simulink model "TestController"  (R2022b)
settings: Solver=FixedStepAuto  StartTime=0.0  StopTime=10.0  RelTol=1e-3
settings Model: Creator=hollis  LastModifiedBy=hollis
settings OptimizationCC: DefaultParameterBehavior=Inlined  EnhancedBackFolding=on  PassReuseOutputArgsAs=Individual arguments  ZeroExternalMemoryAtStartup=off  ZeroInternalMemoryAtStartup=off  OptimizeBlockOrder=speed  DifferentSizesBufferReuse=on  OptimizationCustomize=off  EfficientTunableParamExpr=on
settings DebuggingCC: ParameterTunabilityLossMsg=error
settings SFSimCC: MATLABDynamicMemAlloc=off
settings RTWCC: Description=Embedded Coder  SystemTargetFile=ert.tlc  TemplateMakefile=ert_default_tmf  TargetLang=C++
settings CodeAppCC: ForceParamTrailComments=on  IgnoreCustomStorageClasses=off  OperatorAnnotations=on  SimulinkDataObjDesc=on  SFDataObjDesc=on  InsertBlockDesc=on
settings ERTTargetCC: TargetLangStandard=C++11 (ISO)  GenerateSampleERTMain=on  CodeInterfacePackaging=C++ class  SupportContinuousTime=on  InlinedParameterPlacement=NonHierarchical  RootIOFormat=Structure reference  ERTCustomFileTemplate=example_file_process.tlc

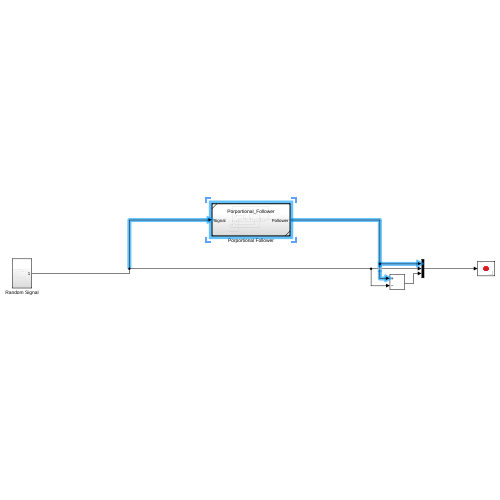
[thumbnail: Simulink's stored preview of the top-level diagram]
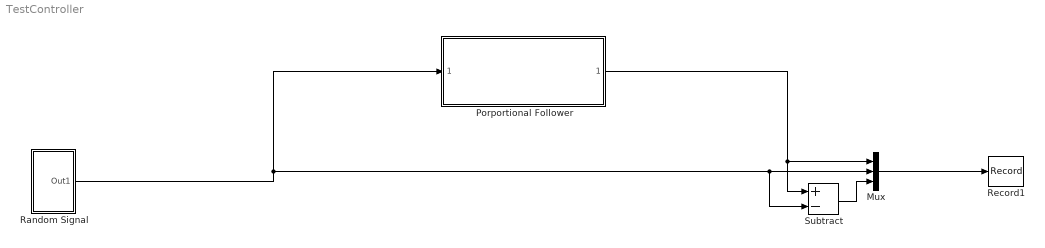
== system TestController ==
  Mux : Mux  Inputs=3
  Porportional Follower : Subsystem  TreatAsAtomicUnit=on  ReferencedSubsystem=Porportional_Follower
  Random Signal : Subsystem
  Record1 : Record  FileSettingsInternal="{\"entries\":[{\"content\":{\"excelSettings\":{\"content\":{},\"type\":\"Streamout.ExcelSettings\"}},\"type\":\"Streamout.FileSettingStorage\",\"uuid\":\"3329fe22-3500-49c1-84ce-a9b356fac455\"}],\"packageUris\":[\"http://schema.mathworks.com/mf0/streamout_blocks/R2020a\"],\"version\":\"1.0\"}"  Layout=[1 1]  SignalsInternal="{\"entries\":[{\"content\":{\"signals\":[{\"content\":{\"blockPath\":[\"TestController/Record1\"],\"channel\":[],\"dimensions\":[3],\"domain\":\"TestController/Record1\",\"hasChildren\":true,\"lineColor\":\"#ff6929\",\"plots\":[],\"port\":1,\"sid\":[\"\"],\"signalID\":55,\"signalName\":\"Mux\"},\"type\":\"RecordBlkView.Signal\",\"uuid\":\"93b944fd-1e56-45a3-8f06-88407ec950c2\"},{\"content\":{\"blockPath\":[\"TestController/Record1\"],\"channel\":[1],\"dimensions\":[3],\"domain\":\"TestController/Record1\",\"lineColor\":\"#fe330a\",\"parentID\":55,\"plots\":[1],\"port\":1,\"sid\":[\"\"],\"signalID\":56,\"signalName\":\"Mux\"},\"type\":\"RecordBlkView.Signal\",\"uuid\":\"28fdb549-0372-403c-af4d-7b99177af04b\"},{\"content\":{\"blockPath\":[\"TestController/Record1\"],\"channel\":[2],\"dimensions\":[3],\"domain\":\"TestController/Record1\",\"lineColor\":\"#22b573\",\"parentID\":55,\"plots\":[1],\"port\":1,\"sid\":[\"\"],\"signalID\":60,\"signalName\":\"Mux\"},\"type\":\"RecordBlkView.Signal\",\"uuid\":\"0bcc67d2-57e9-42fa-b3f9-bc8998f70d9b\"},{\"content\":{\"blockPath\":[\"TestController/Record1\"],\"channel\":[3],\"dimensions\":[3],\"domain\":\"TestController/Record1\",\"lineColor\":\"#b746ff\",\"parentID\":55,\"plots\":[1],\"port\":1,\"sid\":[\"\"],\"signalID\":61,\"signalName\":\"Mux\"},\"type\":\"RecordBlkView.Signal\",\"uuid\":\"bcf16c43-fcd5-4f9a-b691-d8428bd7bb2b\"}]},\"type\":\"RecordBlkView.InputSignals\",\"uuid\":\"c713f41b-1074-4bc9-be1c-7d1e44e526a5\"}],\"packageUris\":[\"http://schema.mathworks.com/mf0/streamout_blocks/R2020a\"],\"version\":\"1.0\"}"  VisualizationBindings="{\"sparklinesplugin\":{\"info\":[{\"bindingParametersList\":[],\"subplotID\":1}]}}"
  Subtract : Sum  Inputs=+-
  wires:
  Random Signal/1(Out1) -> Porportional Follower/1, Subtract/2, Mux/2
  Mux/1 -> Record1/1
  Porportional Follower/1 -> Subtract/1, Mux/1
  Subtract/1 -> Mux/3

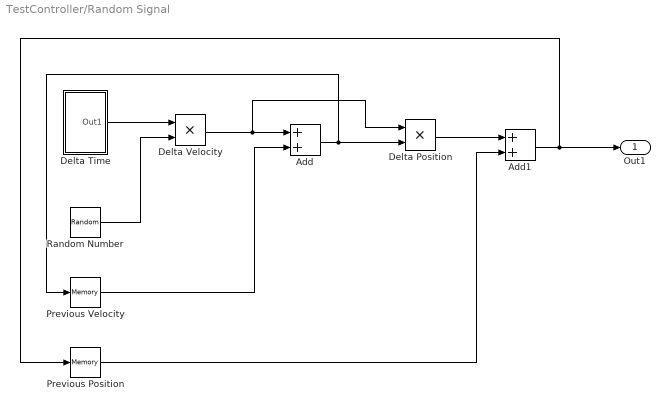
== system TestController/Random Signal ==
  Add : Sum
  Add1 : Sum
  Delta Position : Product
  Delta Time : Subsystem
  Delta Velocity : Product
  Previous Position : Memory
  Previous Velocity : Memory
  Random Number : RandomNumber  Variance=10  Seed=8  SampleTime=0.1
  Out1 : Outport
  wires:
  Previous Position/1 -> Add1/2
  Random Number/1 -> Delta Velocity/2
  Add/1 -> Delta Position/2, Previous Velocity/1
  Delta Position/1 -> Add1/1
  Previous Velocity/1 -> Add/2
  Delta Velocity/1 -> Delta Position/1, Add/1
  Delta Time/1(Out1) -> Delta Velocity/1
  Add1/1 -> Out1/1, Previous Position/1

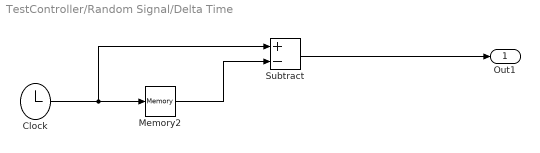
== system TestController/Random Signal/Delta Time ==
  Clock : Clock
  Memory2 : Memory
  Subtract : Sum  Inputs=+-
  Out1 : Outport
  wires:
  Memory2/1 -> Subtract/2
  Clock/1 -> Subtract/1, Memory2/1
  Subtract/1 -> Out1/1
